simulink model "HvCoorn"  (R2022b)
settings: configuration reference "Icar05FusaMdlCfg" (kept outside this file)
undefined symbols (not defined in the file): BMSActSt_ACChrg, BMSActSt_DCChrg, BMSActSt_disconnect, BMSActSt_offline, BMSActSt_online, BMSActSt_undefined, BMSMainNegRlySt_Clsd_SC, BMSMainNegRlySt_Open_SC, BMSMainNegRlySt_StuckInClsd_SC, BMSMainNegRlySt_StuckInOpen_SC, BMSMainPosRlySt_Clsd_SC, BMSMainPosRlySt_Open_SC, BMSMainPosRlySt_StuckInClsd_SC, BMSPrecRlySt_StuckInOpen_SC, BMSReqSt_ACChrg, BMSReqSt_DCChrg, BMSReqSt_emergencyOffline, BMSReqSt_offline, BMSReqSt_online, Chrg_stCycleBookMod_SC, Chrg_stSingleBookMod_SC, CmpgMod_stInactv_SC, DCDCActSt_buck, DCDCActSt_connected, DCDCActSt_disconnected, DCDCReqSt_buck, DCDCReqSt_standby, EngStrtStop_RefuModDft_SC, EPBActSt_Appld_SC, GearLvr_stDrvGearD_SC, GearLvr_stDrvGearN_SC, GearLvr_stDrvGearP_SC, GearLvr_stDrvGearR_SC, hpp_bACChargeLinkIni_C, hpp_bACChargeLinkOKIni_C, hpp_bAcChgEnaIni_C, hpp_bAcChgPauseIni_C, hpp_bAcLinkTempErrIni_C, hpp_bBattWarmReqIni_C, hpp_bHvilHwErrIni_C, hpp_bHvilStOkIni_C, hpp_bHvRelayClsActIni_C, hpp_bHvRelayOpnActIni_C, hpp_bHvRelayStuckIni_C, hpp_bParked4ChDchgIni_C, hpp_bRemLvBatMntnReqIni_C, hpp_bStartUpReqIni_C, hpp_stHvilCanIni_C, hpp_stWarmTimeCfgRespIni_C, HvCoorn_bAuthEnaSwt_C, HvCoorn_bAuthFailSpdLimOvrd_C, HvCoorn_bAuthFailSpdLimOvrdVal_C, HvCoorn_bAuthStrt_C, HvCoorn_bBMSUnexpdDcnctFailEna_C, HvCoorn_bBuck2RdyBypDCDCEna_C, HvCoorn_bDCChrgFctCfg_C, HvCoorn_bDcChrgWkupEnaChrgLink_C, HvCoorn_bDCDcnct4ACEna_C, HvCoorn_bDCNotBuck2ShtdwnEna_C, HvCoorn_bDrvrLevNotRdyEna_C ... (+295)
libraries: ITKLib x213, simulink x61
(part 12 of 12)

== system HvCoorn/HvCoorn/HVP_HighVoltagePowerOnOffProcedure/A30_Authcation/Subsystem1 ==
  HvCoorn_stTboxByte7Fb : Inport
  VCU_Trigger_42C_TX : Inport  Port=2
  Add1 : Sum  Inputs=++++  SaturateOnIntegerOverflow=on
  Add2 : Sum  Inputs=++++  SaturateOnIntegerOverflow=on
  Constant10 : Constant  Value=7
  Constant3 : Constant  Value=0
  Constant4 : Constant
  Constant5 : Constant  Value=2
  Constant6 : Constant  Value=3
  Constant7 : Constant  Value=4
  Constant8 : Constant  Value=5
  Constant9 : Constant  Value=6
  Data Type Conversion{,2..8} (8 alike) : DataTypeConversion  SaturateOnIntegerOverflow=off  RndMeth=Floor
  Gain : Gain  OutDataTypeStr=uint8
  Gain1 : Gain  Gain=2  OutDataTypeStr=uint8
  Gain2 : Gain  Gain=4  OutDataTypeStr=uint8
  Gain3 : Gain  Gain=8  OutDataTypeStr=uint8
  Gain4 : Gain  OutDataTypeStr=uint8
  Gain5 : Gain  Gain=2  OutDataTypeStr=uint8
  Gain6 : Gain  Gain=4  OutDataTypeStr=uint8
  Gain7 : Gain  Gain=8  OutDataTypeStr=uint8
  Saturation : Saturate  UpperLimit=15  LowerLimit=0
  Saturation1 : Saturate  UpperLimit=15  LowerLimit=0
  Subsystem{1..8} (8 alike) : ITKLib/BitOperation/Subsystem1
      settings: SourceProductName=ITKC_Lib
  Switch1 : Switch  Criteria=u2 ~= 0  SaturateOnIntegerOverflow=off  InputSameDT=off
      settings: AttributesFormatString=Criteria : %<Criteria>
  Switch11 : Switch  Criteria=u2 ~= 0  SaturateOnIntegerOverflow=off  InputSameDT=off
      settings: AttributesFormatString=Criteria : %<Criteria>
  TaskTime_s2 : Constant  Value=TaskTime_10ms
      settings: AttributesFormatString=[0.01]
  Turn_Off_Delay_Vari1 : ITKLib/TimeCounter/Turn_Off_Delay_Vari
      settings: AttributesFormatString=TurnOffDelay  SourceProductName=ITKC_Lib
  sup_tiChgConndown_C : Constant  Description=[3]  Value=HvCoorn_ti430triggerDly_C
      settings: AttributesFormatString=%<Description>
  uint1 : Constant  Value=0  OutDataTypeStr=uint8  SampleTime=-1
      settings: AttributesFormatString=%<OutDataTypeStr>
  uint5 : Constant  Value=0  OutDataTypeStr=uint8  SampleTime=-1
      settings: AttributesFormatString=%<OutDataTypeStr>
  TBOX_receiver_module_FB : Outport  VectorParamsAs1DForOutWhenUnconnected=off
  TBOX_Instruction_Type_FB : Outport  Port=2  VectorParamsAs1DForOutWhenUnconnected=off
  wires:
  Constant7/1 -> Subsystem5/1
  Constant10/1 -> Subsystem8/1
  Constant4/1 -> Subsystem2/1
  Constant9/1 -> Subsystem7/1
  HvCoorn_stTboxByte7Fb/1 -> Subsystem1/2, Subsystem2/2, Subsystem3/2, Subsystem8/2, Subsystem7/2, Subsystem6/2, Subsystem5/2, Subsystem4/2
  Constant3/1 -> Subsystem1/1
  Constant8/1 -> Subsystem6/1
  Data Type Conversion7/1 -> Gain2/1
  Constant5/1 -> Subsystem3/1
  Constant6/1 -> Subsystem4/1
  Data Type Conversion5/1 -> Gain/1
  Gain3/1 -> Add1/4
  Gain/1 -> Add1/1
  Gain2/1 -> Add1/3
  Gain1/1 -> Add1/2
  Data Type Conversion8/1 -> Gain3/1
  Data Type Conversion6/1 -> Gain1/1
  Subsystem2/1 -> Data Type Conversion2/1
  Subsystem4/1 -> Data Type Conversion4/1
  Gain5/1 -> Add2/2
  Gain6/1 -> Add2/3
  Gain4/1 -> Add2/1
  Gain7/1 -> Add2/4
  Subsystem1/1 -> Data Type Conversion/1
  Subsystem3/1 -> Data Type Conversion3/1
  Switch1/1 -> TBOX_receiver_module_FB/1  "TBOX_receiver_module_FB"
  Add2/1 -> Saturation/1
  Add1/1 -> Saturation1/1
  Data Type Conversion/1 -> Gain4/1
  Data Type Conversion2/1 -> Gain5/1
  Data Type Conversion3/1 -> Gain6/1
  Data Type Conversion4/1 -> Gain7/1
  Subsystem5/1 -> Data Type Conversion5/1
  Subsystem8/1 -> Data Type Conversion8/1
  Subsystem7/1 -> Data Type Conversion7/1
  Subsystem6/1 -> Data Type Conversion6/1
  Turn_Off_Delay_Vari1/1 -> Switch11/2, [VCU_Trigger_42Cdly_TX]
  uint5/1 -> Switch11/3
  [VCU_Trigger_42Cdly_TX] -> Switch1/2
  uint1/1 -> Switch1/3
  Switch11/1 -> TBOX_Instruction_Type_FB/1  "TBOX_Instruction_Type_FB"
  Saturation1/1 -> Switch1/1
  Saturation/1 -> Switch11/1
  TaskTime_s2/1 -> Turn_Off_Delay_Vari1/2
  sup_tiChgConndown_C/1 -> Turn_Off_Delay_Vari1/3
  VCU_Trigger_42C_TX/1 -> Turn_Off_Delay_Vari1/1

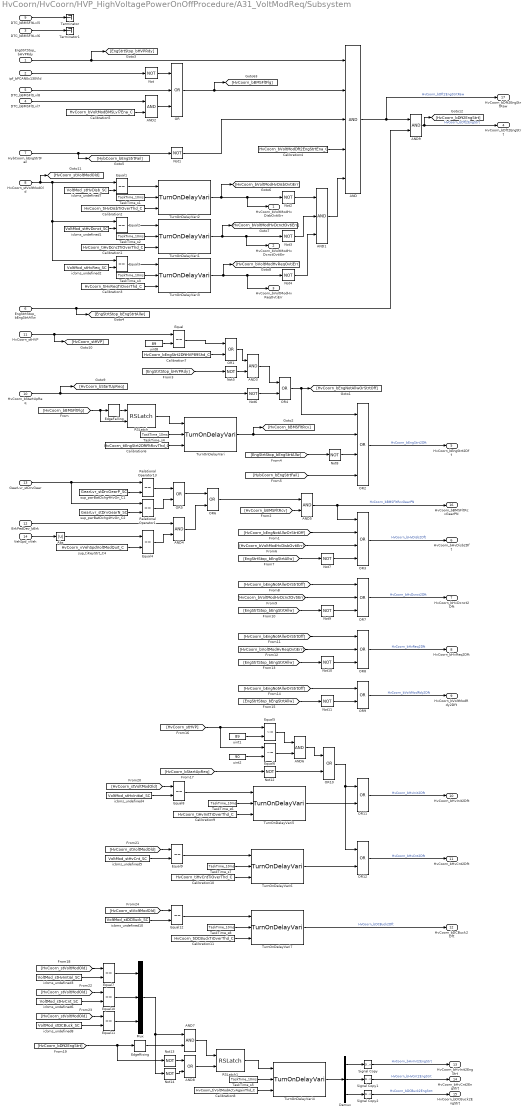
== system HvCoorn/HvCoorn/HVP_HighVoltagePowerOnOffProcedure/A31_VoltModReq/Subsystem ==
  EngStrtStop_bHVPRdy : Inport
  ipf_bPCAN0x130Vld : Inport  Port=2
  DTC_bBMSFltLvl6 : Inport  Port=3
  DTC_bBMSFltLvl7 : Inport  Port=4
  DTC_bBMSFltLvl8 : Inport  Port=5
  EngStrtStop_bEngStrtAllw : Inport  Port=6
  HybCoorn_bEngStrtFail : Inport  Port=7
  HvCoorn_stVoltModOld : Inport  Port=8
  DTC_bBMSFltLvl5 : Inport  Port=9
  HvCoorn_bStartUpReq : Inport  Port=10
  HvCoorn_stHVP : Inport  Port=11
  BrkPedDev_bBrk : Inport  Port=12
  GearLvr_stDrvGear : Inport  Port=13
  VehSpd_vVeh : Inport  Port=14
  AND : Logic  Inputs=5  OutDataTypeStr=boolean
  AND1 : Logic  Inputs=3  OutDataTypeStr=boolean
  AND{2..7,9} (7 alike) : Logic  OutDataTypeStr=boolean
  AND8 : Logic  Operator=OR  OutDataTypeStr=boolean
  Abs : Abs  SaturateOnIntegerOverflow=off  OutDataTypeStr=Inherit: Inherit via internal rule
  Calibration1 : Constant  Description=[5]  Value=HvCoorn_tiHvDcnctTiOverThd_C  SampleTime=-1
      settings: AttributesFormatString=%<Description>
  Calibration10 : Constant  Description=[5]  Value=HvCoorn_tiHvCntTiOverThd_C  SampleTime=-1
      settings: AttributesFormatString=%<Description>
  Calibration11 : Constant  Description=[0.1]  Value=HvCoorn_tiDCBuckTiOverThd_C  SampleTime=-1
      settings: AttributesFormatString=%<Description>
  Calibration2 : Constant  Description=[5]  Value=HvCoorn_tiHvDisbTiOverThd_C  SampleTime=-1
      settings: AttributesFormatString=%<Description>
  Calibration3 : Constant  Description=[5]  Value=HvCoorn_tiHvReqTiOverThd_C  SampleTime=-1
      settings: AttributesFormatString=%<Description>
  Calibration4 : Constant  Description=[0]  Value=HvCoorn_bVoltModDft2EngStrtEna_C  SampleTime=-1
      settings: AttributesFormatString=%<Description>
  Calibration5 : Constant  Description=[0]  Value=HvCoorn_bVoltModBMSLvl7Ena_C  SampleTime=-1
      settings: AttributesFormatString=%<Description>
  Calibration6 : Constant  Description=[1]  Value=HvCoorn_tiEngStrt2DftFltRcvThd_C  SampleTime=-1
      settings: AttributesFormatString=%<Description>
  Calibration7 : Constant  Description=[0]  Value=HvCoorn_bEngStrt2DftHVP89Shd_C  SampleTime=-1
      settings: AttributesFormatString=%<Description>
  Calibration8 : Constant  Description=[1]  Value=HvCoorn_tiVoltModActvAgainThd_C  SampleTime=-1
      settings: AttributesFormatString=%<Description>
  Calibration9 : Constant  Description=[5]  Value=HvCoorn_tiHvInitTiOverThd_C  SampleTime=-1
      settings: AttributesFormatString=%<Description>
  Demux : Demux  Outputs=3
  EdgeFalling : ITKLib/Memory/EdgeFalling  Tag=initial value = 0
      settings: SourceProductName=ITKC_Lib
  EdgeRising : ITKLib/Memory/EdgeRising  Tag=initial value = 0
      settings: SourceProductName=ITKC_Lib
  Equal : RelationalOperator  Operator===  OutDataTypeStr=boolean  RndMeth=Simplest  InputSameDT=off
  Equal{1..3,7..12} (9 alike) : RelationalOperator  Operator===  OutDataTypeStr=boolean
  Equal4 : RelationalOperator  Operator=<=  OutDataTypeStr=boolean  RndMeth=Simplest  InputSameDT=off
  Equal5 : RelationalOperator  Operator=~=  OutDataTypeStr=boolean  RndMeth=Simplest  InputSameDT=off
  Equal6 : RelationalOperator  Operator=~=  OutDataTypeStr=boolean  RndMeth=Simplest  InputSameDT=off
  Mux : Mux  Inputs=3
  Not{,1..14} (15 alike) : Logic  Operator=NOT  AllPortsSameDT=off  OutDataTypeStr=boolean
  OR : Logic  Operator=OR  Inputs=3  OutDataTypeStr=boolean
  OR{1,4..6,9..12} (8 alike) : Logic  Operator=OR  OutDataTypeStr=boolean
  OR2 : Logic  Operator=OR  Inputs=4  OutDataTypeStr=boolean
  OR3 : Logic  Operator=OR  Inputs=4  OutDataTypeStr=boolean
  OR7 : Logic  Operator=OR  Inputs=3  OutDataTypeStr=boolean
  OR8 : Logic  Operator=OR  Inputs=3  OutDataTypeStr=boolean
  RSLatch : ITKLib/Memory/RSLatch
      settings: SourceProductName=ITKC_Lib
  RSLatch1 : ITKLib/Memory/RSLatch
      settings: SourceProductName=ITKC_Lib
  Relational Operator1 : RelationalOperator  Operator===  OutDataTypeStr=boolean  InputSameDT=off
  Relational Operator13 : RelationalOperator  Operator===  OutDataTypeStr=boolean  InputSameDT=off
  Signal Copy : SignalConversion  OverrideOpt=off
  Signal Copy1 : SignalConversion  OverrideOpt=off
  Signal Copy2 : SignalConversion  OverrideOpt=off
  TaskTime_s{1..8} (8 alike) : Constant  Value=TaskTime_10ms
      settings: AttributesFormatString=[0.01]
  Terminator : Terminator
  Terminator1 : Terminator
  TurnOnDelayVari{,1..7} (8 alike) : ITKLib/TimeCounter/TurnOnDelayVari
      settings: AttributesFormatString=TurnOnDelay  SourceProductName=ITKC_Lib
  icbms_undefined1 : Constant  Description=[3]  Value=VoltMod_stHvDcnct_SC  OutDataTypeStr=uint8
      settings: AttributesFormatString=%<Description>
  icbms_undefined10 : Constant  Description=[8]  Value=VoltMod_stDCBuck_SC  OutDataTypeStr=uint8
      settings: AttributesFormatString=%<Description>
  icbms_undefined2 : Constant  Description=[4]  Value=VoltMod_stHvReq_SC  OutDataTypeStr=uint8
      settings: AttributesFormatString=%<Description>
  icbms_undefined3 : Constant  Description=[6]  Value=VoltMod_stHvInitial_SC  OutDataTypeStr=uint8
      settings: AttributesFormatString=%<Description>
  icbms_undefined4 : Constant  Description=[6]  Value=VoltMod_stHvInitial_SC  OutDataTypeStr=uint8
      settings: AttributesFormatString=%<Description>
  icbms_undefined5 : Constant  Description=[7]  Value=VoltMod_stHvCnt_SC  OutDataTypeStr=uint8
      settings: AttributesFormatString=%<Description>
  icbms_undefined6 : Constant  Description=[7]  Value=VoltMod_stHvCnt_SC  OutDataTypeStr=uint8
      settings: AttributesFormatString=%<Description>
  icbms_undefined7 : Constant  Description=[2]  Value=VoltMod_stHvDisb_SC  OutDataTypeStr=uint8
      settings: AttributesFormatString=%<Description>
  icbms_undefined8 : Constant  Description=[8]  Value=VoltMod_stDCBuck_SC  OutDataTypeStr=uint8
      settings: AttributesFormatString=%<Description>
  sup_pwrBatDchg4HvOn_C1 : Constant  Description=[6]  Value=GearLvr_stDrvGearP_SC
      settings: AttributesFormatString=%<Description>
  sup_pwrBatDchg4HvOn_C2 : Constant  Description=[4]  Value=GearLvr_stDrvGearN_SC
      settings: AttributesFormatString=%<Description>
  sup_tiKeyStrt_C4 : Constant  Description=[3]  Value=HvCoorn_vVehSpdVoltModQuit_C
      settings: AttributesFormatString=%<Description>
  uint1 : Constant  Value=89  OutDataTypeStr=uint8  SampleTime=-1
      settings: AttributesFormatString=%<OutDataTypeStr>
  uint2 : Constant  Value=90  OutDataTypeStr=uint8  SampleTime=-1
      settings: AttributesFormatString=%<OutDataTypeStr>
  uint8 : Constant  Value=89  OutDataTypeStr=uint8  SampleTime=-1
      settings: AttributesFormatString=%<OutDataTypeStr>
  HvCoorn_bVoltModHvDisbOvtiErr : Outport  VectorParamsAs1DForOutWhenUnconnected=off
  HvCoorn_bVoltModHvDcnctOvtiErr : Outport  Port=2  VectorParamsAs1DForOutWhenUnconnected=off
  HvCoorn_bVoltModHvReqOvtiErr : Outport  Port=3  VectorParamsAs1DForOutWhenUnconnected=off
  HvCoorn_bDft2EngStrt : Outport  Port=4  VectorParamsAs1DForOutWhenUnconnected=off
  HvCoorn_bEngStrt2Dft : Outport  Port=5  VectorParamsAs1DForOutWhenUnconnected=off
  HvCoorn_bHvDisb2Dft : Outport  Port=6  VectorParamsAs1DForOutWhenUnconnected=off
  HvCoorn_bHvDcnct2Dft : Outport  Port=7  VectorParamsAs1DForOutWhenUnconnected=off
  HvCoorn_bHvReq2Dft : Outport  Port=8  VectorParamsAs1DForOutWhenUnconnected=off
  HvCoorn_bVoltModRdy2Dft : Outport  Port=9  VectorParamsAs1DForOutWhenUnconnected=off
  HvCoorn_bHvInit2Dft : Outport  Port=10  VectorParamsAs1DForOutWhenUnconnected=off
  HvCoorn_bHvCnt2Dft : Outport  Port=11  VectorParamsAs1DForOutWhenUnconnected=off
  HvCoorn_bDCBuck2Dft : Outport  Port=12  VectorParamsAs1DForOutWhenUnconnected=off
  HvCoorn_bHvInit2EngStrt : Outport  Port=13  VectorParamsAs1DForOutWhenUnconnected=off
  HvCoorn_bHvCnt2EngStrt : Outport  Port=14  VectorParamsAs1DForOutWhenUnconnected=off
  HvCoorn_bDCBuck2EngStrt : Outport  Port=15  VectorParamsAs1DForOutWhenUnconnected=off
  HvCoorn_bBMSFltRcvGearPN : Outport  Port=16  VectorParamsAs1DForOutWhenUnconnected=off
  HvCoorn_bDft2EngStrtRaw : Outport  Port=17  VectorParamsAs1DForOutWhenUnconnected=off
  wires:
  Not1/1 -> AND/3
  OR/1 -> [HvCoorn_bBMSFltFlg], AND/2
  AND9/1 -> [HvCoorn_bDft2EngStrt], HvCoorn_bDft2EngStrt/1  "HvCoorn_bDft2EngStrt"
  ipf_bPCAN0x130Vld/1 -> Not/1
  Not/1 -> OR/1
  HvCoorn_stVoltModOld/1 -> [HvCoorn_stVoltModOld], Equal3/1, Equal2/1, Equal1/1
  icbms_undefined7/1 -> Equal1/2
  icbms_undefined1/1 -> Equal2/2
  icbms_undefined2/1 -> Equal3/2
  Calibration2/1 -> TurnOnDelayVari2/3
  TaskTime_s1/1 -> TurnOnDelayVari2/2
  Equal1/1 -> TurnOnDelayVari2/1
  TaskTime_s2/1 -> TurnOnDelayVari1/2
  Calibration1/1 -> TurnOnDelayVari1/3
  Equal2/1 -> TurnOnDelayVari1/1
  Calibration3/1 -> TurnOnDelayVari3/3
  TaskTime_s3/1 -> TurnOnDelayVari3/2
  Equal3/1 -> TurnOnDelayVari3/1
  TurnOnDelayVari2/1 -> HvCoorn_bVoltModHvDisbOvtiErr/1, Not2/1, [HvCoorn_bVoltModHvDisbOvtiErr]
  TurnOnDelayVari1/1 -> [HvCoorn_bVoltModHvDcnctOvtiErr], HvCoorn_bVoltModHvDcnctOvtiErr/1, Not3/1
  TurnOnDelayVari3/1 -> [HvCoorn_bVoltModHvReqOvtiErr], HvCoorn_bVoltModHvReqOvtiErr/1, Not4/1
  Not2/1 -> AND1/1
  Not3/1 -> AND1/2
  Not4/1 -> AND1/3
  AND1/1 -> AND/5
  DTC_bBMSFltLvl8/1 -> OR/2
  Calibration4/1 -> AND/4
  AND2/1 -> OR/3
  DTC_bBMSFltLvl7/1 -> AND2/1
  Calibration5/1 -> AND2/2
  Not6/1 -> OR4/2
  TurnOnDelayVari/1 -> [HvCoorn_bBMSFltRcv], OR2/2
  [HvCoorn_bBMSFltFlg] -> RSLatch/2, EdgeFalling/1
  Not5/1 -> AND3/2
  Calibration6/1 -> TurnOnDelayVari/3
  HvCoorn_bStartUpReq/1 -> [HvCoorn_bStartUpReq], Not6/1
  Equal/1 -> OR1/1
  TaskTime_s4/1 -> TurnOnDelayVari/2
  OR2/1 -> HvCoorn_bEngStrt2Dft/1  "HvCoorn_bEngStrt2Dft"
  AND3/1 -> OR4/1
  uint8/1 -> Equal/2
  OR1/1 -> AND3/1
  HvCoorn_stHVP/1 -> [HvCoorn_stHVP], Equal/1
  Calibration7/1 -> OR1/2
  OR3/1 -> HvCoorn_bHvDisb2Dft/1  "HvCoorn_bHvDisb2Dft"
  Not8/1 -> OR2/3
  OR4/1 -> [HvCoorn_bEngNotAllwOrStrtOff], OR2/1
  [HvCoorn_bEngNotAllwOrStrtOff] -> OR3/2
  EdgeFalling/1 -> RSLatch/1
  RSLatch/1 -> TurnOnDelayVari/1
  sup_tiKeyStrt_C4/1 -> Equal4/2
  sup_pwrBatDchg4HvOn_C1/1 -> Relational Operator13/2
  GearLvr_stDrvGear/1 -> Relational Operator1/1, Relational Operator13/1
  VehSpd_vVeh/1 -> Abs/1
  sup_pwrBatDchg4HvOn_C2/1 -> Relational Operator1/2
  Relational Operator1/1 -> OR5/2
  Relational Operator13/1 -> OR5/1
  OR5/1 -> OR6/1
  BrkPedDev_bBrk/1 -> AND4/1
  Equal4/1 -> AND4/2
  AND4/1 -> OR6/2
  OR6/1 -> AND5/1
  [HvCoorn_bBMSFltRcv] -> AND5/2
  AND5/1 -> HvCoorn_bBMSFltRcvGearPN/1, OR3/1  "HvCoorn_bBMSFltRcvGearPN"
  EngStrtStop_bHVPRdy/1 -> [EngStrtStop_bHVPRdy], AND/1
  [EngStrtStop_bHVPRdy] -> Not5/1
  HybCoorn_bEngStrtFail/1 -> [HybCoorn_bEngStrtFail], Not1/1
  EngStrtStop_bEngStrtAllw/1 -> AND9/2, [EngStrtStop_bEngStrtAllw]
  [EngStrtStop_bEngStrtAllw] -> Not8/1
  [HybCoorn_bEngStrtFail] -> OR2/4
  [HvCoorn_bVoltModHvDisbOvtiErr] -> OR3/3
  [EngStrtStop_bEngStrtAllw] -> Not7/1
  Not7/1 -> OR3/4
  OR7/1 -> HvCoorn_bHvDcnct2Dft/1  "HvCoorn_bHvDcnct2Dft"
  [HvCoorn_bEngNotAllwOrStrtOff] -> OR7/1
  [HvCoorn_bVoltModHvDcnctOvtiErr] -> OR7/2
  [EngStrtStop_bEngStrtAllw] -> Not9/1
  Not9/1 -> OR7/3
  [HvCoorn_bEngNotAllwOrStrtOff] -> OR8/1
  [HvCoorn_bVoltModHvReqOvtiErr] -> OR8/2
  [EngStrtStop_bEngStrtAllw] -> Not10/1
  Not10/1 -> OR8/3
  OR8/1 -> HvCoorn_bHvReq2Dft/1  "HvCoorn_bHvReq2Dft"
  OR9/1 -> HvCoorn_bVoltModRdy2Dft/1  "HvCoorn_bVoltModRdy2Dft"
  [HvCoorn_bEngNotAllwOrStrtOff] -> OR9/1
  [EngStrtStop_bEngStrtAllw] -> Not11/1
  Not11/1 -> OR9/2
  uint1/1 -> Equal5/2
  [HvCoorn_stHVP] -> Equal6/1, Equal5/1
  uint2/1 -> Equal6/2
  Equal5/1 -> AND6/1
  Equal6/1 -> AND6/2
  Not12/1 -> OR10/2
  [HvCoorn_bStartUpReq] -> Not12/1
  AND6/1 -> OR10/1
  OR11/1 -> HvCoorn_bHvInit2Dft/1  "HvCoorn_bHvInit2Dft"
  icbms_undefined3/1 -> Equal7/2
  [HvCoorn_stVoltModOld] -> Equal7/1
  RSLatch1/1 -> TurnOnDelayVari4/1
  EdgeRising/1 -> AND7/2
  Calibration8/1 -> TurnOnDelayVari4/3
  TaskTime_s5/1 -> TurnOnDelayVari4/2
  [HvCoorn_bDft2EngStrt] -> Not13/1, EdgeRising/1
  Not13/1 -> AND8/1
  AND7/1 -> RSLatch1/1
  [HvCoorn_stVoltModOld] -> Equal8/1
  icbms_undefined4/1 -> Equal8/2
  TaskTime_s6/1 -> TurnOnDelayVari5/2
  Calibration9/1 -> TurnOnDelayVari5/3
  Equal8/1 -> TurnOnDelayVari5/1
  TurnOnDelayVari5/1 -> OR11/2
  OR10/1 -> OR12/1, OR11/1
  OR12/1 -> HvCoorn_bHvCnt2Dft/1  "HvCoorn_bHvCnt2Dft"
  Equal9/1 -> TurnOnDelayVari6/1
  Calibration10/1 -> TurnOnDelayVari6/3
  TaskTime_s7/1 -> TurnOnDelayVari6/2
  icbms_undefined5/1 -> Equal9/2
  [HvCoorn_stVoltModOld] -> Equal9/1
  TurnOnDelayVari6/1 -> OR12/2
  Equal7/1 -> Mux/1
  Mux/1 -> AND7/1, Not14/1
  [HvCoorn_stVoltModOld] -> Equal10/1
  icbms_undefined6/1 -> Equal10/2
  Equal10/1 -> Mux/2
  icbms_undefined8/1 -> Equal11/2
  [HvCoorn_stVoltModOld] -> Equal11/1
  Equal11/1 -> Mux/3
  TurnOnDelayVari4/1 -> Demux/1
  Demux/1 -> Signal Copy/1
  Demux/2 -> Signal Copy1/1
  Demux/3 -> Signal Copy2/1
  Signal Copy/1 -> HvCoorn_bHvInit2EngStrt/1  "HvCoorn_bHvInit2EngStrt"
  Signal Copy1/1 -> HvCoorn_bHvCnt2EngStrt/1  "HvCoorn_bHvCnt2EngStrt"
  Signal Copy2/1 -> HvCoorn_bDCBuck2EngStrt/1  "HvCoorn_bDCBuck2EngStrt"
  [HvCoorn_stVoltModOld] -> Equal12/1
  icbms_undefined10/1 -> Equal12/2
  TaskTime_s8/1 -> TurnOnDelayVari7/2
  Calibration11/1 -> TurnOnDelayVari7/3
  Equal12/1 -> TurnOnDelayVari7/1
  TurnOnDelayVari7/1 -> HvCoorn_bDCBuck2Dft/1  "HvCoorn_bDCBuck2Dft"
  Abs/1 -> Equal4/1
  AND8/1 -> RSLatch1/2
  Not14/1 -> AND8/2
  DTC_bBMSFltLvl5/1 -> Terminator/1
  DTC_bBMSFltLvl6/1 -> Terminator1/1
  AND/1 -> HvCoorn_bDft2EngStrtRaw/1, AND9/1  "HvCoorn_bDft2EngStrtRaw"

== system HvCoorn/HvCoorn/HVP_HighVoltagePowerOnOffProcedure/A31_VoltModReq/Subsystem1 ==
  icems_stEng : Inport
  ved_bInhbEngStrt : Inport  Port=2
  icems_nAct : Inport  Port=3
  AND : Logic  Inputs=3  OutDataTypeStr=boolean
  AND1 : Logic  OutDataTypeStr=boolean
  Calibration1 : Constant  Description=[0.5]  Value=HvCoorn_tiEngStrt2HvDisbThd_C  SampleTime=-1
      settings: AttributesFormatString=%<Description>
  Not : Logic  Operator=NOT  AllPortsSameDT=off  OutDataTypeStr=boolean
  Relational Operator1 : RelationalOperator  OutDataTypeStr=boolean
      settings: DeleteFcn=if exist('delete_tlblock','file')==2,delete_tlblock(gcbh);end  NameChangeFcn=if exist('rename_tlblock','file')==2,rename_tlblock(gcbh);end  OpenFcn=if exist('tl_open_blockdlg','file')==2,tl_open_blockdlg(gcbh);else,open_system(gcbh,'parameter');end
  Relational Operator4 : RelationalOperator  Operator=<=  OutDataTypeStr=boolean
      settings: DeleteFcn=if exist('delete_tlblock','file')==2,delete_tlblock(gcbh);end  NameChangeFcn=if exist('rename_tlblock','file')==2,rename_tlblock(gcbh);end  OpenFcn=if exist('tl_open_blockdlg','file')==2,tl_open_blockdlg(gcbh);else,open_system(gcbh,'parameter');end
  Relational Operator6 : RelationalOperator  Operator===  OutDataTypeStr=boolean
      settings: DeleteFcn=if exist('delete_tlblock','file')==2,delete_tlblock(gcbh);end  NameChangeFcn=if exist('rename_tlblock','file')==2,rename_tlblock(gcbh);end  OpenFcn=if exist('tl_open_blockdlg','file')==2,tl_open_blockdlg(gcbh);else,open_system(gcbh,'parameter');end
  TaskTime_s3 : Constant  Value=TaskTime_10ms
      settings: AttributesFormatString=[0.01]
  TurnOnDelayVari1 : ITKLib/TimeCounter/TurnOnDelayVari
      settings: AttributesFormatString=TurnOnDelay  SourceProductName=ITKC_Lib
  icemsSt_Run_SC1 : Constant  Description=[1100]  Value=HvCoorn_nEngStrt2HvDisbUppr_C  OutDataTypeStr=Inherit: Inherit via back propagation  SampleTime=-1
      settings: AttributesFormatString=%<Description>  CopyFcn=if exist('tl_reset_reviewflag','file')==2,tl_reset_reviewflag(gcbh);end  DeleteFcn=if exist('delete_tlblock','file')==2,delete_tlblock(gcbh);end  NameChangeFcn=if exist('rename_tlblock','file')==2,rename_tlblock(gcbh);end  OpenFcn=if exist('tl_open_blockdlg','file')==2,tl_open_blockdlg(gcbh);else,open_system(gcbh,'parameter');end
  icemsSt_Run_SC2 : Constant  Description=[3]  Value=icems_stEngRun_SC  OutDataTypeStr=Inherit: Inherit via back propagation  SampleTime=-1
      settings: AttributesFormatString=%<Description>  CopyFcn=if exist('tl_reset_reviewflag','file')==2,tl_reset_reviewflag(gcbh);end  DeleteFcn=if exist('delete_tlblock','file')==2,delete_tlblock(gcbh);end  NameChangeFcn=if exist('rename_tlblock','file')==2,rename_tlblock(gcbh);end  OpenFcn=if exist('tl_open_blockdlg','file')==2,tl_open_blockdlg(gcbh);else,open_system(gcbh,'parameter');end
  icemsSt_Run_SC3 : Constant  Description=[900]  Value=HvCoorn_nEngStrt2HvDisbLowr_C  OutDataTypeStr=Inherit: Inherit via back propagation  SampleTime=-1
      settings: AttributesFormatString=%<Description>  CopyFcn=if exist('tl_reset_reviewflag','file')==2,tl_reset_reviewflag(gcbh);end  DeleteFcn=if exist('delete_tlblock','file')==2,delete_tlblock(gcbh);end  NameChangeFcn=if exist('rename_tlblock','file')==2,rename_tlblock(gcbh);end  OpenFcn=if exist('tl_open_blockdlg','file')==2,tl_open_blockdlg(gcbh);else,open_system(gcbh,'parameter');end
  HvCoorn_bEngStrt2HvDisb : Outport  VectorParamsAs1DForOutWhenUnconnected=off
  wires:
  icemsSt_Run_SC2/1 -> Relational Operator6/2
  icems_stEng/1 -> Relational Operator6/1
  Relational Operator6/1 -> AND/1
  ved_bInhbEngStrt/1 -> Not/1
  Not/1 -> AND/2
  icemsSt_Run_SC1/1 -> Relational Operator4/2
  icems_nAct/1 -> Relational Operator1/1, Relational Operator4/1
  Relational Operator4/1 -> AND1/1
  Relational Operator1/1 -> AND1/2
  icemsSt_Run_SC3/1 -> Relational Operator1/2
  AND1/1 -> AND/3
  TaskTime_s3/1 -> TurnOnDelayVari1/2
  Calibration1/1 -> TurnOnDelayVari1/3
  AND/1 -> TurnOnDelayVari1/1
  TurnOnDelayVari1/1 -> HvCoorn_bEngStrt2HvDisb/1  "HvCoorn_bEngStrt2HvDisb"

== system HvCoorn/HvCoorn/HVP_HighVoltagePowerOnOffProcedure/A31_VoltModReq/Subsystem2 ==
  icbms_stMainPosRly : Inport
  icbms_stMainNegRly : Inport  Port=2
  icbms_iHVBat : Inport  Port=3
  HvCoorn_stVoltModOld : Inport  Port=4
  AND : Logic  OutDataTypeStr=boolean
  Calibration2 : Constant  Description=[0.03]  Value=HvCoorn_tiHvDisb2HvDcnctThd_C  SampleTime=-1
      settings: AttributesFormatString=%<Description>
  Equal1 : RelationalOperator  Operator===  OutDataTypeStr=boolean
  OR : Logic  Operator=OR  OutDataTypeStr=boolean
  OR1 : Logic  Operator=OR  OutDataTypeStr=boolean
  Relational Operator1 : RelationalOperator  Operator===  OutDataTypeStr=boolean  InputSameDT=off
  Relational Operator2 : RelationalOperator  Operator=<  OutDataTypeStr=boolean
      settings: DeleteFcn=if exist('delete_tlblock','file')==2,delete_tlblock(gcbh);end  NameChangeFcn=if exist('rename_tlblock','file')==2,rename_tlblock(gcbh);end  OpenFcn=if exist('tl_open_blockdlg','file')==2,tl_open_blockdlg(gcbh);else,open_system(gcbh,'parameter');end
  Relational Operator8 : RelationalOperator  Operator===  OutDataTypeStr=boolean  InputSameDT=off
  TaskTime_s1 : Constant  Value=TaskTime_10ms
      settings: AttributesFormatString=[0.01]
  TurnOnDelayVari2 : ITKLib/TimeCounter/TurnOnDelayVari
      settings: AttributesFormatString=TurnOnDelay  SourceProductName=ITKC_Lib
  icbms_undefined1 : Constant  Description=[2]  Value=VoltMod_stHvDisb_SC  OutDataTypeStr=uint8
      settings: AttributesFormatString=%<Description>
  icbms_undefined7 : Constant  Description=[1]  Value=BMSMainNegRlySt_Open_SC  OutDataTypeStr=uint8
      settings: AttributesFormatString=%<Description>
  icbms_undefined8 : Constant  Description=[1]  Value=BMSMainPosRlySt_Open_SC  OutDataTypeStr=uint8
      settings: AttributesFormatString=%<Description>
  icemsSt_Run_SC3 : Constant  Description=[5]  Value=HvCoorn_iHvBatHvDisb2HvDcnctThd_C  OutDataTypeStr=Inherit: Inherit via back propagation  SampleTime=-1
      settings: AttributesFormatString=%<Description>  CopyFcn=if exist('tl_reset_reviewflag','file')==2,tl_reset_reviewflag(gcbh);end  DeleteFcn=if exist('delete_tlblock','file')==2,delete_tlblock(gcbh);end  NameChangeFcn=if exist('rename_tlblock','file')==2,rename_tlblock(gcbh);end  OpenFcn=if exist('tl_open_blockdlg','file')==2,tl_open_blockdlg(gcbh);else,open_system(gcbh,'parameter');end
  HvCoorn_bHvDisb2HvDcnct : Outport  VectorParamsAs1DForOutWhenUnconnected=off
  HvCoorn_bHvDcnct2HvReq : Outport  Port=2  VectorParamsAs1DForOutWhenUnconnected=off
  wires:
  icbms_stMainNegRly/1 -> Relational Operator1/1
  icbms_stMainPosRly/1 -> Relational Operator8/1
  icbms_undefined8/1 -> Relational Operator8/2
  icbms_undefined7/1 -> Relational Operator1/2
  Relational Operator8/1 -> OR/1
  Relational Operator1/1 -> OR/2
  Calibration2/1 -> TurnOnDelayVari2/3
  TaskTime_s1/1 -> TurnOnDelayVari2/2
  icemsSt_Run_SC3/1 -> Relational Operator2/2
  icbms_iHVBat/1 -> Relational Operator2/1
  OR/1 -> HvCoorn_bHvDcnct2HvReq/1, OR1/1  "HvCoorn_bHvDcnct2HvReq"
  TurnOnDelayVari2/1 -> OR1/2
  OR1/1 -> HvCoorn_bHvDisb2HvDcnct/1  "HvCoorn_bHvDisb2HvDcnct"
  HvCoorn_stVoltModOld/1 -> Equal1/1
  icbms_undefined1/1 -> Equal1/2
  Relational Operator2/1 -> AND/2
  Equal1/1 -> AND/1
  AND/1 -> TurnOnDelayVari2/1

== system HvCoorn/HvCoorn/HVP_HighVoltagePowerOnOffProcedure/A31_VoltModReq/Subsystem3 ==
  icfm_uAct : Inport
  icrm_uAct : Inport  Port=2
  icisg_uAct : Inport  Port=3
  icisg_stMod : Inport  Port=4
  AND : Logic  OutDataTypeStr=boolean
  Calibration3 : Constant  Description=[1]  Value=HvCoorn_tiHvReq2VoltModRdyThd_C  SampleTime=-1
      settings: AttributesFormatString=%<Description>
  Equal1 : RelationalOperator  Operator===  OutDataTypeStr=boolean
  MinMax : MinMax  Function=max  Inputs=3  SaturateOnIntegerOverflow=on
  Relational Operator7 : RelationalOperator  Operator=>  OutDataTypeStr=boolean  InputSameDT=off
  TaskTime_s3 : Constant  Value=TaskTime_10ms
      settings: AttributesFormatString=[0.01]
  TurnOnDelayVari3 : ITKLib/TimeCounter/TurnOnDelayVari
      settings: AttributesFormatString=TurnOnDelay  SourceProductName=ITKC_Lib
  sup_uIpuShutdown_C : Constant  Description=[220]  Value=HvCoorn_uMax4VoltModRdy_C
      settings: AttributesFormatString=%<Description>
  uint8 : Constant  Value=4  OutDataTypeStr=uint8  SampleTime=-1
      settings: AttributesFormatString=%<OutDataTypeStr>
  HvCoorn_bHvReq2VoltModRdy : Outport  VectorParamsAs1DForOutWhenUnconnected=off
  wires:
  icfm_uAct/1 -> MinMax/1
  icrm_uAct/1 -> MinMax/2
  icisg_uAct/1 -> MinMax/3
  sup_uIpuShutdown_C/1 -> Relational Operator7/2
  MinMax/1 -> Relational Operator7/1
  Relational Operator7/1 -> AND/1
  icisg_stMod/1 -> Equal1/1
  Equal1/1 -> AND/2
  uint8/1 -> Equal1/2  "Volt_Control"
  TurnOnDelayVari3/1 -> HvCoorn_bHvReq2VoltModRdy/1  "HvCoorn_bHvReq2VoltModRdy"
  TaskTime_s3/1 -> TurnOnDelayVari3/2
  Calibration3/1 -> TurnOnDelayVari3/3
  AND/1 -> TurnOnDelayVari3/1

== system HvCoorn/HvCoorn/HVP_HighVoltagePowerOnOffProcedure/A31_VoltModReq/Subsystem4 ==
  HvCoorn_bStartUpReq : Inport
  HvCoorn_stHVP : Inport  Port=2
  HvCoorn_bBMSFltRcvGearPN : Inport  Port=3
  icfm_stMode : Inport  Port=4
  icrm_stMode : Inport  Port=5
  icdc_stMode : Inport  Port=6
  icisg_stMod : Inport  Port=7
  VehCfg_bFrntMotByp : Inport  Port=8
  HvGrid_pwrLoadAct : Inport  Port=9
  icfm_uAct : Inport  Port=10
  icdc_uHvAct : Inport  Port=11
  icrm_uAct : Inport  Port=12
  AND : Logic  Inputs=3  OutDataTypeStr=boolean
  AND1 : Logic  Inputs=5  OutDataTypeStr=boolean
  AND2 : Logic  OutDataTypeStr=boolean
  AND3 : Logic  OutDataTypeStr=boolean
  Constant1 : Constant  Description=[2]  Value=MCUActSt_standby
      settings: AttributesFormatString=[2]
  Constant3 : Constant  Description=[2]  Value=MCUActSt_standby
      settings: AttributesFormatString=[2]
  Equal{,1..6} (7 alike) : RelationalOperator  Operator===  OutDataTypeStr=boolean  RndMeth=Simplest  InputSameDT=off
  Equal7 : RelationalOperator  Operator=<  OutDataTypeStr=boolean  RndMeth=Simplest  InputSameDT=off
  Min : MinMax  Function=max  Inputs=3  InputSameDT=on  SaturateOnIntegerOverflow=on
  OR : Logic  Operator=OR  OutDataTypeStr=boolean
  OR1 : Logic  Operator=OR  OutDataTypeStr=boolean
  OR2 : Logic  Operator=OR  OutDataTypeStr=boolean
  Relational Operator1 : RelationalOperator  OutDataTypeStr=boolean  InputSameDT=off
  sup_tiKeyStrt_C4 : Constant  Description=[500]  Value=HvCoorn_pwrLoadActHvInit2HvCnt_C
      settings: AttributesFormatString=%<Description>
  sup_uThres_C : Constant  Description=[220]  Value=HvCoorn_uThd4HvCnt2DCBuck_C
      settings: AttributesFormatString=%<Description>
  uint1 : Constant  Value=90  OutDataTypeStr=uint8  SampleTime=-1
      settings: AttributesFormatString=%<OutDataTypeStr>
  uint2 : Constant  Value=2  OutDataTypeStr=uint8  SampleTime=-1
      settings: AttributesFormatString=%<OutDataTypeStr>
  uint3 : Constant  OutDataTypeStr=uint8  SampleTime=-1
      settings: AttributesFormatString=%<OutDataTypeStr>
  uint5 : Constant  Value=2  OutDataTypeStr=uint8  SampleTime=-1
      settings: AttributesFormatString=%<OutDataTypeStr>
  uint8 : Constant  Value=89  OutDataTypeStr=uint8  SampleTime=-1
      settings: AttributesFormatString=%<OutDataTypeStr>
  HvCoorn_bHvDcnct2HvInit : Outport  VectorParamsAs1DForOutWhenUnconnected=off
  HvCoorn_bHvInit2HvCnt : Outport  Port=2  VectorParamsAs1DForOutWhenUnconnected=off
  HvCoorn_bHvCnt2DCBuck : Outport  Port=3  VectorParamsAs1DForOutWhenUnconnected=off
  wires:
  HvCoorn_bBMSFltRcvGearPN/1 -> AND/3
  AND/1 -> AND3/1, AND2/1, HvCoorn_bHvDcnct2HvInit/1  "HvCoorn_bHvDcnct2HvInit"
  uint8/1 -> Equal/2
  HvCoorn_stHVP/1 -> Equal1/1, Equal/1
  Equal1/1 -> OR2/2
  HvCoorn_bStartUpReq/1 -> AND/2
  OR2/1 -> AND/1
  Equal/1 -> OR2/1
  uint1/1 -> Equal1/2
  Constant1/1 -> Equal2/2
  icfm_stMode/1 -> Equal2/1
  Constant3/1 -> Equal3/2
  icrm_stMode/1 -> Equal3/1
  Equal2/1 -> OR/1
  VehCfg_bFrntMotByp/1 -> OR/2
  icdc_stMode/1 -> Equal4/1
  uint2/1 -> Equal4/2
  icisg_stMod/1 -> Equal6/1, Equal5/1
  uint3/1 -> Equal5/2
  uint5/1 -> Equal6/2
  Equal5/1 -> OR1/1
  Equal6/1 -> OR1/2
  OR/1 -> AND1/1
  OR1/1 -> AND1/4
  HvGrid_pwrLoadAct/1 -> Equal7/1
  sup_tiKeyStrt_C4/1 -> Equal7/2
  Equal3/1 -> AND1/2
  Equal4/1 -> AND1/3
  Equal7/1 -> AND1/5
  AND1/1 -> AND2/2
  AND2/1 -> HvCoorn_bHvInit2HvCnt/1  "HvCoorn_bHvInit2HvCnt"
  AND3/1 -> HvCoorn_bHvCnt2DCBuck/1  "HvCoorn_bHvCnt2DCBuck"
  Min/1 -> Relational Operator1/1
  icfm_uAct/1 -> Min/1
  icdc_uHvAct/1 -> Min/3
  icrm_uAct/1 -> Min/2
  sup_uThres_C/1 -> Relational Operator1/2
  Relational Operator1/1 -> AND3/2

== stateflow chart HvCoorn/HVP_HighVoltagePowerOnOffProcedure/A30_Authcation/Auth_status ==
  settings: updateMethod=DISCRETE
  state init
    en:
    authfailed_n_conter=authfailed_n_conterEER;
    auth_enum=uint8(0);
  state Wait
    en:
    auth_enum=uint8(1);
  state ISO
    en:
    timer= uint8(0);
    auth_enum=uint8(4);
    du:
    authfailed_n_conterEEW=authfailed_n_conter;
    timer= timer+1;
    state Counter
      en:
      authfailed_n_conter=authfailed_n_conter+1;
    (default) -> Counter
  state Equal
    en:
    auth_enum=uint8(2);
    timer= uint8(0);
    authfailed_n_conter= TCP_AnomalyOfAntitheftCheck;
    du:
    authfailed_n_conterEEW=authfailed_n_conter;
    timer= timer+1;
  state Reset
    en:
    auth_enum=uint8(3);
    timer= uint8(0);
    authfailed_n_conter= uint8(0);
    du:
    authfailed_n_conterEEW=authfailed_n_conter;
    timer= timer+1;
  (default) -> init
  init -> Wait : [Hvcoorn_bEEReadOver]
  Equal -> Wait : [timer>=10]
  Wait -> ISO [order 2] : [authfailed||VCCM_flg_Antitheft_Overtime]
  Wait -> Equal [order 3] : [fault_counterequal]
  Reset -> Wait [order 2] : [timer>=10]
  Wait -> Reset [order 1] : [authsuccess||HvCoorn_bClearZero]
  ISO -> Wait [order 1] : [timer>=10]
  ISO -> Reset [order 2] : [authsuccess||HvCoorn_bClearZero]
  Reset -> ISO [order 1] : [authfailed||VCCM_flg_Antitheft_Overtime]
  data: authfailed_n_conterEEW output uint8; authsuccess input boolean; authfailed_n_conter output uint8; authfailed input boolean; authfailed_n_conterEER input uint8; VCCM_flg_Antitheft_Overtime input boolean; HvCoorn_bClearZero input boolean; fault_counterequal input boolean; timer local double; TCP_AnomalyOfAntitheftCheck input uint8; auth_enum output uint8; Hvcoorn_bEEReadOver input boolean

== stateflow chart HvCoorn/HVP_HighVoltagePowerOnOffProcedure/A19_MainProcedure ==
  state WakeUp
    en:
    HvCoorn_stHVP = uint8(1);
  state VcuPowerShutDown
    en:
    HvCoorn_stHVP = uint8(130);
  state NmHoldState
    en:
    HvCoorn_stHVP = uint8(125);
  state Initial_Settings
    en:
    HvCoorn_stHVP = uint8(10);
  state VcuAfterRun
    en:
    HvCoorn_stHVP = uint8(121);
  state Normal
    state Startup
      state Wait4Communication
        en:
        HvCoorn_stHVP = uint8(11);
      state HvContactorRequest
        en:
        HvCoorn_stHVP = uint8(12);
      state DCDCBuckReq
        en:
        HvCoorn_stHVP = uint8(17);
      (default) -> Wait4Communication
      Wait4Communication -> HvContactorRequest [order 1] : [HvCoorn_bComm2HVReq]
      HvContactorRequest -> DCDCBuckReq [order 1] : [HvCoorn_bHVReq2DCBuck]
    state Shutdown
      state Shutdown_OthersECU
        en:
        HvCoorn_stHVP = uint8(115);
      state Shutdown_HV
        en:
        HvCoorn_stHVP = uint8(101);
      state Shutdown_DisChErr
        en:
        HvCoorn_stHVP = uint8(110);
      state Shutdown_MotDischarge
        en:
        HvCoorn_stHVP = uint8(105);
      (default) -> Shutdown_HV
      Shutdown_MotDischarge -> Shutdown_OthersECU [order 1] : [HvCoorn_bShutDisCh2ShutECU]
      Shutdown_DisChErr -> Shutdown_OthersECU : [after(1,tick)]
      Shutdown_HV -> Shutdown_MotDischarge : [HvCoorn_bShutHV2ShutDisCh]
      Shutdown_MotDischarge -> Shutdown_DisChErr [order 2] : [HvCoorn_bShutDisCh2ShutErr]
    state HVReady
      state Wait4MindChange
        en:
        HvCoorn_stHVP = uint8(95);
      state Wait4ComMindChange
        en:
        HvCoorn_stHVP = uint8(91);
      state SystemReady
        state SystemReadyWait
          en:
          HvCoorn_stHVP = uint8(89);
        state SystemReady
          en:
          HvCoorn_stHVP = uint8(90);
        (default) -> SystemReadyWait
        Normal.HVReady.SystemReady.SystemReady -> SystemReadyWait : [HvCoorn_bRdy2RdyWait]
        SystemReadyWait -> Normal.HVReady.SystemReady.SystemReady : [HvCoorn_bRdyWait2Rdy]
      (default) -> Wait4MindChange
      Wait4MindChange -> Wait4ComMindChange [order 2] : [HvCoorn_bStartUpReq]
      Wait4ComMindChange -> Wait4MindChange [order 1] : [!HvCoorn_bStartUpReq]
      Normal.HVReady.SystemReady -> Wait4MindChange : [!HvCoorn_bStartUpReq && HvCoorn_bVehSpd4HvDown && HvCoorn_bAPUNotRdy]
      Wait4ComMindChange -> Normal.HVReady.SystemReady [order 2] : [HvCoorn_bMindChag2Rdy]
    (default) -> Startup
    Shutdown_OthersECU -> Startup [order 2] : [HvCoorn_bShutECU2Comm]
    Wait4Communication -> Shutdown_OthersECU [order 2] : [HvCoorn_bComm2ShutECU]
    HvContactorRequest -> Shutdown [order 2] : [HvCoorn_bHVReq2ShutDown]
    Wait4MindChange -> Shutdown_HV [order 1] : [HvCoorn_bMindChag2ShutHV]
    DCDCBuckReq -> Shutdown [order 2] : [HvCoorn_bDCBuck2Shtdwn]
    DCDCBuckReq -> Normal.HVReady.SystemReady [order 1] : [HvCoorn_bDCBuck2Rdy ]
  state Emergency_HV
    state Emergency_ShutDownIni
      en:
      HvCoorn_stHVP = uint8(151);
    state Emergency_ShutdownHV
      en:
      HvCoorn_stHVP = uint8(152);
    state Emergency_MotDischarge
      en:
      HvCoorn_stHVP = uint8(154);
    state Emergency_DisChErr
      en:
      HvCoorn_stHVP = uint8(155);
    state Emergency_Wait4KeyOff
      en:
      HvCoorn_stHVP = uint8(156);
    state Emergency_NmHoldState
      en:
      HvCoorn_stHVP = uint8(158);
    state Emergency_VcuPowerShutDown
      en:
      HvCoorn_stHVP = uint8(160);
    (default) -> Emergency_ShutDownIni
    Emergency_ShutDownIni -> Emergency_ShutdownHV : [HvCoorn_bEmIni2ShutHV]
    Emergency_ShutdownHV -> Emergency_MotDischarge : [HvCoorn_bEmShutHv2DisCh]
    Emergency_MotDischarge -> Emergency_DisChErr [order 1] : [HvCoorn_bEmDisCh2Err]
    Emergency_MotDischarge -> Emergency_Wait4KeyOff [order 2] : [HvCoorn_bEmDisCh2WaitKeyOff]
    Emergency_DisChErr -> Emergency_Wait4KeyOff : [after(1,tick)]
    Emergency_Wait4KeyOff -> Emergency_NmHoldState : [HvCoorn_bEmWaitKeyOff2NetMan]
    Emergency_NmHoldState -> Emergency_VcuPowerShutDown : [HvCoorn_bNetMan2PwrShut]
  (default) -> WakeUp
  VcuPowerShutDown -> WakeUp : [HvCoorn_bStartUpReq]
  NmHoldState -> VcuPowerShutDown [order 2] : [HvCoorn_bNetMan2PwrShut]
  WakeUp -> NmHoldState [order 2] : [HvCoorn_bWake2NetMan]
  NmHoldState -> WakeUp [order 1] : [HvCoorn_bStartUpReq]
  VcuAfterRun -> NmHoldState [order 2] : [HvCoorn_bAftRun2NetMan]
  WakeUp -> Initial_Settings [order 1] : [HvCoorn_bStartUpReq&&after(2,tick)]
  Emergency_HV -> Initial_Settings : [HvCoorn_bEmShutHeal]
  VcuAfterRun -> Initial_Settings [order 1] : [HvCoorn_bStartUpReq]
  Initial_Settings -> VcuAfterRun [order 2] : [HvCoorn_bInit2AftRun]
  Initial_Settings -> Startup [order 1] : [HvCoorn_bInit2StrtUp]
  Shutdown_OthersECU -> VcuAfterRun [order 1] : [HvCoorn_bShutECU2AftRun]
  Normal -> Emergency_HV : [HvCoorn_bEmgcyShutDownReq]
  data: HvCoorn_bStartUpReq input boolean; HvCoorn_stHVP output uint8 =0; HvCoorn_bInit2StrtUp input boolean; HvCoorn_bComm2HVReq input boolean; HvCoorn_bComm2ShutECU input boolean; HvCoorn_bHVReq2DCBuck input boolean; HvCoorn_bHVReq2ShutDown input boolean; HvCoorn_bDCBuck2Rdy input boolean; HvCoorn_bDCBuck2Shtdwn input boolean; HvCoorn_bRdyWait2Rdy input boolean; HvCoorn_bRdy2RdyWait input boolean; HvCoorn_bMindChag2Rdy input boolean; HvCoorn_bMindChag2ShutHV input boolean; HvCoorn_bShutHV2ShutDisCh input boolean; HvCoorn_bShutDisCh2ShutECU input boolean; HvCoorn_bShutDisCh2ShutErr input boolean; HvCoorn_bShutECU2AftRun input boolean; HvCoorn_bShutECU2Comm input boolean; HvCoorn_bAftRun2NetMan input boolean; HvCoorn_bNetMan2PwrShut input boolean; HvCoorn_bWake2NetMan input boolean; HvCoorn_bInit2AftRun input boolean; HvCoorn_bEmIni2ShutHV input boolean; HvCoorn_bEmShutHv2DisCh input boolean; HvCoorn_bEmDisCh2WaitKeyOff input boolean; HvCoorn_bEmDisCh2Err input boolean; HvCoorn_bEmWaitKeyOff2NetMan input boolean; HvCoorn_bEmShutHeal input boolean; HvCoorn_bEmgcyShutDownReq input boolean; HvCoorn_bVehSpd4HvDown input; HvCoorn_bAPUNotRdy input boolean

== stateflow chart HvCoorn/HVP_HighVoltagePowerOnOffProcedure/A32_VoltModSts ==
  state Default
    en:
    HvCoorn_stVoltMod=VoltMod_stDft_SC;%0
    HvCoorn_bVoltModStbReq=boolean(0);
  state EngStrt
    en:
    HvCoorn_stVoltMod=VoltMod_stEngStrt_SC;%1
    HvCoorn_bVoltModStbReq=boolean(0);
  state HvDisb
    en:
    HvCoorn_stVoltMod=VoltMod_stHvDisb_SC;%2
    HvCoorn_bVoltModStbReq=boolean(1);
  state VoltMod
    state HvDcnct
      en:
      HvCoorn_stVoltMod=VoltMod_stHvDcnct_SC;%3
      HvCoorn_bVoltModStbReq=boolean(1);
    state HvReq
      en:
      HvCoorn_stVoltMod=VoltMod_stHvReq_SC;%4
      HvCoorn_bVoltModStbReq=boolean(1);
    state VoltModRdy
      en:
      HvCoorn_stVoltMod=VoltMod_stVoltModRdy_SC;%5
      HvCoorn_bVoltModStbReq=boolean(0);
    (default) -> HvDcnct
    HvDcnct -> HvReq [order 1] : [HvCoorn_bHvDcnct2HvReq]
    HvReq -> VoltModRdy [order 1] : [HvCoorn_bHvReq2VoltModRdy]
  state HvInitial
    en:
    HvCoorn_stVoltMod=VoltMod_stHvInitial_SC;%6
    HvCoorn_bVoltModStbReq=boolean(1);
  state HvCnt
    en:
    HvCoorn_stVoltMod=VoltMod_stHvCnt_SC;%7
    HvCoorn_bVoltModStbReq=boolean(1);
  state DCDCBuck
    en:
    HvCoorn_stVoltMod=VoltMod_stDCBuck_SC;%8
    HvCoorn_bVoltModStbReq=boolean(1);
  (default) -> Default
  Default -> EngStrt : [HvCoorn_bDft2EngStrt]
  EngStrt -> Default [order 2] : [HvCoorn_bEngStrt2Dft]
  HvDisb -> Default [order 2] : [HvCoorn_bHvDisb2Dft]
  HvDcnct -> Default [order 2] : [HvCoorn_bHvDcnct2Dft]
  HvReq -> Default [order 2] : [HvCoorn_bHvReq2Dft]
  VoltModRdy -> Default : [HvCoorn_bVoltModRdy2Dft]
  HvInitial -> Default [order 2] : [HvCoorn_bHvInit2Dft]
  HvCnt -> Default [order 2] : [HvCoorn_bHvCnt2Dft]
  DCDCBuck -> Default [order 1] : [HvCoorn_bDCBuck2Dft]
  DCDCBuck -> EngStrt [order 2] : [HvCoorn_bDCBuck2EngStrt]
  HvCnt -> EngStrt [order 3] : [HvCoorn_bHvCnt2EngStrt]
  HvInitial -> EngStrt [order 3] : [HvCoorn_bHvInit2EngStrt]
  EngStrt -> HvDisb [order 1] : [HvCoorn_bEngStrt2HvDisb]
  HvDisb -> HvDcnct [order 1] : [HvCoorn_bHvDisb2HvDcnct]
  VoltMod -> HvInitial : [HvCoorn_bHvDcnct2HvInit]
  HvInitial -> HvCnt [order 1] : [HvCoorn_bHvInit2HvCnt]
  HvCnt -> DCDCBuck [order 1] : [HvCoorn_bHvCnt2DCBuck]
  data: HvCoorn_bDft2EngStrt input boolean; HvCoorn_bEngStrt2HvDisb input boolean; HvCoorn_bHvDisb2HvDcnct input boolean; HvCoorn_bHvDcnct2HvReq input boolean; HvCoorn_bHvReq2VoltModRdy input boolean; HvCoorn_stVoltMod output uint8; VoltMod_stDft_SC constant uint8 =VoltMod_stDft_SC; VoltMod_stEngStrt_SC constant uint8 =VoltMod_stEngStrt_SC; VoltMod_stHvDisb_SC constant uint8 =VoltMod_stHvDisb_SC; VoltMod_stHvDcnct_SC constant uint8 =VoltMod_stHvDcnct_SC; VoltMod_stHvReq_SC constant uint8 =VoltMod_stHvReq_SC; VoltMod_stVoltModRdy_SC constant uint8 =VoltMod_stVoltModRdy_SC; HvCoorn_bVoltModStbReq output boolean; VoltMod_stHvInitial_SC constant uint8 =VoltMod_stHvInitial_SC; VoltMod_stHvCnt_SC constant uint8 =VoltMod_stHvCnt_SC; VoltMod_stDCBuck_SC constant uint8 =VoltMod_stDCBuck_SC; HvCoorn_bEngStrt2Dft input boolean; HvCoorn_bHvDisb2Dft input boolean; HvCoorn_bHvDcnct2Dft input boolean; HvCoorn_bHvReq2Dft input boolean; HvCoorn_bVoltModRdy2Dft input boolean; HvCoorn_bHvInit2Dft input boolean; HvCoorn_bHvCnt2Dft input boolean; HvCoorn_bDCBuck2Dft input boolean; HvCoorn_bHvDcnct2HvInit input boolean; HvCoorn_bHvInit2HvCnt input boolean; HvCoorn_bHvCnt2DCBuck input boolean; HvCoorn_bHvInit2EngStrt input boolean; HvCoorn_bHvCnt2EngStrt input boolean; HvCoorn_bDCBuck2EngStrt input boolean
